simulink model "celsius_to_fahrenheit_conversion"  (R2019b)
settings: Solver=VariableStepAuto  StartTime=0.0  StopTime=10.0  RelTol=1e-3
undefined symbols (not defined in the file): X
settings Model: Creator=46769  LastModifiedBy=46769
settings DebuggingCC: SFMachineParentedDataDiag=error

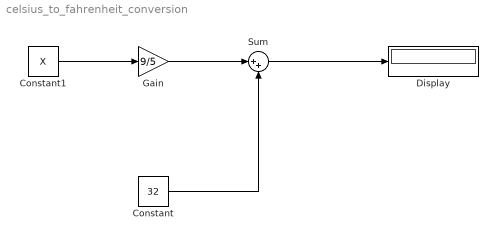
== system celsius_to_fahrenheit_conversion ==
  Constant : Constant  Value=32
  Constant1 : Constant  Value=X
  Display : Display
  Gain : Gain  Gain=9/5
  Sum : Sum  Inputs=|++
  wires:
  Gain/1 -> Sum/1
  Constant/1 -> Sum/2
  Sum/1 -> Display/1
  Constant1/1 -> Gain/1
